simulink model "wind_turbine_power_sim"  (R2022b)
settings: Solver=FixedStepAuto  StartTime=0.0  StopTime=20  FixedStep=0.01  RelTol=1e-3
undefined symbols (not defined in the file or in its folder): ratedPower
settings Model: Creator=randy  LastModifiedBy=randy

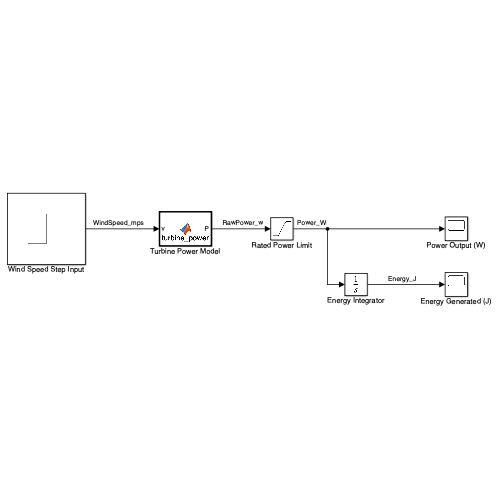
[thumbnail: Simulink's stored preview of the top-level diagram]
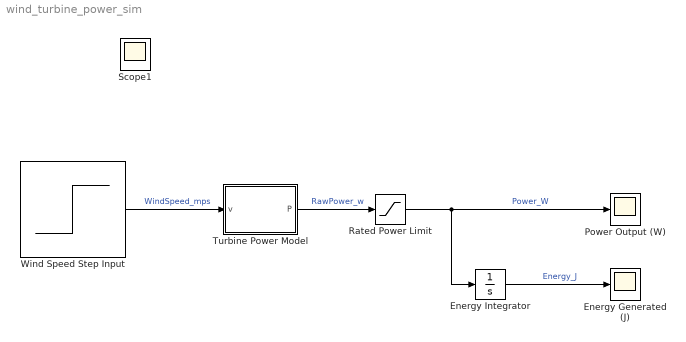
== system wind_turbine_power_sim ==
  Energy Generated (J) : Scope
  Energy Integrator : Integrator
  Power Output (W) : Scope
  Rated Power Limit : Saturate  UpperLimit=ratedPower  LowerLimit=0
  Turbine Power Model : MATLAB Function  TreatAsAtomicUnit=on
  Wind Speed Step Input : Step  Time=2  Before=5  After=15  SampleTime=0
  Scope1 : Scope
  wires:
  Wind Speed Step Input/1 -> Turbine Power Model/1(v)  "WindSpeed_mps"
  Turbine Power Model/1(P) -> Rated Power Limit/1  "RawPower_w"
  Rated Power Limit/1 -> Power Output (W)/1, Energy Integrator/1  "Power_W"
  Energy Integrator/1 -> Energy Generated (J)/1  "Energy_J"

== matlab function wind_turbine_power_sim/Turbine Power Model ==
  data: v input; P output
function P = turbine_power(v)
% Simplified wind turbine power model
% v = wind speed in m/s
% P = output power in watts

rho = 1.225;
bladeRadius = 1.5;
A = pi * bladeRadius^2;
Cp = 0.35;

cutIn = 3;
cutOut = 25;

if v < cutIn
    P = 0;
elseif v > cutOut
    P = 0;
else
    P = 0.5 * rho * A * Cp * v^3;
end
